simulink model "VTOLAutopilotController"  (R2025a)
settings: configuration reference "VTOLConfiguration" (kept outside this file)
undefined symbols (not defined in the file): Back_Transition_Rate, const, control, controlParams, ControlSampleTime, CriticalTiltAngle, DiscIntNeverNeededParam, dspblkCoreblockFVToolHelper, Fading_time, flightState, FSState, FWControlParams, FWTrimSpeed, gcbh, HoverMission, ReferenceFilterDen, ReferenceFilterNum, tilt_max, tiltIni, TransitioncontrolGains, uavParam, uavParams, VTOLcontrolGains, w_trim, WindDownRate
libraries: simulink x43, slpidlib x35, uavalgslib x7, simulink_extras x1
(part 2 of 8)

== system VTOLAutopilotController/Low level controller/Scheduler/Subsystem ==
  note: Multicopter Control Mixer
  note: MotorCommand1 : commanded phi torque (roll)
      | MotorCommand2 : commanded theta torque (pitch)
      | MotorCommand3 : commanded psi torque (yaw)
      | MotorCommand4 : commaned thrust
      | MotorCommand5 : command tilt
  FlightState : Inport
  FixedWingActuators : Inport  Port=2
  MotorCommands : Inport  Port=3
  TiltSchedule : Inport  Port=4
  TransitionDone : Inport  Port=5
  States : Inport  Port=6
  Actuator To Voltage : Subsystem
  Bus Selector1 : BusSelector  OutputSignals=Vb
  Merge : Merge  Inputs=4
  Scope{,1..3} (4 alike) : Scope
      Scope settings: ActiveDisplayYMinimum=-3975.75811  ActiveDisplayYMaximum=34801.34103  DataLoggingVariableName=ScopeData3
      Scope1 settings: ActiveDisplayYMinimum=0.5844  ActiveDisplayYMaximum=0.95477  DataLoggingVariableName=ScopeData4
      Scope2 settings: ActiveDisplayYMinimum=0.36457  ActiveDisplayYMaximum=0.73494  DataLoggingVariableName=ScopeData5
      Scope3 settings: ActiveDisplayYMinimum=0.36457  ActiveDisplayYMaximum=0.73494  DataLoggingVariableName=ScopeData6
  Switch Case : SwitchCase  CaseConditions={flightState.Hover, flightState.Transition, flightState.FixedWing,flightState.BackTransition}  ShowDefaultCase=off
  Switch Case Action Subsystem : Subsystem  TreatAsAtomicUnit=on
  Switch Case Action Subsystem1 : Subsystem  TreatAsAtomicUnit=on
  Switch Case Action Subsystem2 : Subsystem  TreatAsAtomicUnit=on
  Switch Case Action Subsystem3 : Subsystem  TreatAsAtomicUnit=on
  To Workspace : ToWorkspace  VariableName=Body_Velocity  SaveFormat=Timeseries  SampleTime=-1
  ActuatorControls : Outport  OutDataTypeStr=Bus: RotorCtrlBus
  wires:
  Merge/1 -> Scope/1, Actuator To Voltage/1(Motor Commands)
  Switch Case/4 -> Switch Case Action Subsystem3/Action
  MotorCommands/1 -> Switch Case Action Subsystem3/1(MixerCommands), Scope2/1, Switch Case Action Subsystem/1(MixerCommands), Switch Case Action Subsystem1/2(MixerCommands)
  States/1 -> Switch Case Action Subsystem1/5(State), Switch Case Action Subsystem2/3(State), Bus Selector1/1
  Switch Case Action Subsystem2/1(Actuator) -> Merge/3
  Switch Case Action Subsystem/1(Actuator) -> Merge/1
  Switch Case Action Subsystem3/1(Actuator) -> Merge/4
  FixedWingActuators/1 -> Switch Case Action Subsystem3/3(FixedWing), Switch Case Action Subsystem2/1(FixedWingCtrlBus), Switch Case Action Subsystem1/3(FixedWing)
  Switch Case/3 -> Switch Case Action Subsystem2/Action
  TransitionDone/1 -> Switch Case Action Subsystem1/4(TransitionDone), Switch Case Action Subsystem2/2(TransitionDone)
  Actuator To Voltage/1(To PWM) -> Scope1/1, ActuatorControls/1
  Switch Case/2 -> Switch Case Action Subsystem1/Action
  Switch Case Action Subsystem1/1(Actuator) -> Merge/2
  TiltSchedule/1 -> Switch Case Action Subsystem1/1(TiltSchedule), Switch Case Action Subsystem3/2(TiltSchedule)
  Switch Case/1 -> Switch Case Action Subsystem/Action
  Bus Selector1/1 -> To Workspace/1, Scope3/1  "<Vb>"
  FlightState/1 -> Switch Case/1

== system VTOLAutopilotController/Low level controller/Tilt Scheduler/Back Transition Scheduler ==
  Tilt Schedule : Inport
  FlightMode : Inport  Port=2
  States : Inport  Port=3
  Add : Sum  Commented=on  Inputs=+-
  Bus Selector : BusSelector  Commented=on  OutputSignals=Vb
  Constant1 : Constant  Value=flightState.BackTransition
  Constant2 : Constant  Value=0
  Constant5 : Constant  Value=-Back_Transition_Rate
  Constant6 : Constant  Commented=on  Value=4
  Discrete-Time Integrator : DiscreteIntegrator  ExternalReset=rising  InitialConditionSource=external  SampleTime=-1  LimitOutput=on  UpperSaturationLimit=pi/2  LowerSaturationLimit=0  ICPrevOutput=DiscIntNeverNeededParam  ICPrevScaledInput=DiscIntNeverNeededParam
  Equal : RelationalOperator  Operator===  OutDataTypeStr=boolean  RndMeth=Simplest  InputSameDT=off
  Saturation : Saturate  Commented=on  UpperLimit=pi/4  LowerLimit=-pi/4
  Selector : Selector  Commented=on  InputPortWidth=3  IndexOptions=Index vector (dialog)  Indices=[1]  OutputSizes=1
  Switch1 : Switch  Criteria=u2 > Threshold  SaturateOnIntegerOverflow=off  InputSameDT=off
  Switch2 : Switch  Threshold=1  SaturateOnIntegerOverflow=off  InputSameDT=off
  Vx Controller : slpidlib/PID Controller  Commented=on  Controller=P  Form=Parallel  TimeDomain=Discrete-time  UseExternalTs=off  SampleTime=0.005  IntegratorMethod=Forward Euler  FilterMethod=Forward Euler  ControllerParametersSource=internal  P=controlParams.P_BACK  I=0  UseKiTs=off  D=0.0379422021775223  UseExternalDerivativeSource=off  N=1.96946409823213  UseFilter=on  TunerSelectOption=Transfer Function Based (PID Tuner App)  InitialConditionSource=internal  InitialConditionForIntegrator=0  InitialConditionForFilter=0  DifferentiatorICPrevScaledInput=0  ExternalReset=none  TrackingMode=off  Kt=1  LimitOutput=off  SatLimitsSource=internal  UpperSaturationLimit=inf  LowerSaturationLimit=-inf  LinearizeAsGain=on  AntiWindupMode=none  Kb=1  LimitIntegrator=off  UpperIntegratorSaturationLimit=inf  LowerIntegratorSaturationLimit=-inf  POutMin=[]  POutMax=[]  IOutMin=[]  IOutMax=[]  DOutMin=[]  DOutMax=[]  NOutMin=[]  NOutMax=[]  SumOutMin=[]  SumOutMax=[]  SaturationOutMin=[]  SaturationOutMax=[]  PParamMin=[]  PParamMax=[]  IParamMin=[]  IParamMax=[]  DParamMin=[]  DParamMax=[]  NParamMin=[]  NParamMax=[]  KbParamMin=[]  KbParamMax=[]  KtParamMin=[]  KtParamMax=[]  KbOutMin=[]  KbOutMax=[]  KtOutMin=[]  KtOutMax=[]  IntegratorOutMin=[]  IntegratorOutMax=[]  FilterOutMin=[]  FilterOutMax=[]  SumI1OutMin=[]  SumI1OutMax=[]  SumI2OutMin=[]  SumI2OutMax=[]  SumI3OutMin=[]  SumI3OutMax=[]  SumI4OutMin=[]  SumI4OutMax=[]  SumDOutMin=[]  SumDOutMax=[]  DifferentiatorOutMin=[]  DifferentiatorOutMax=[]  FilterDiffOutCoefMin=[]  FilterDiffOutCoefMax=[]  ReciprocalOutMin=[]  ReciprocalOutMax=[]  SumDenOutMin=[]  SumDenOutMax=[]  SumNumOutMin=[]  SumNumOutMax=[]  DivideOutMin=[]  DivideOutMax=[]  UdiffTsProdOutMin=[]  UdiffTsProdOutMax=[]  NTsProdOutMin=[]  NTsProdOutMax=[]  UintegralTsProdOutMin=[]  UintegralTsProdOutMax=[]  UngainTsProdOutMin=[]  UngainTsProdOutMax=[]  ClampingZeroOutDataTypeStr=Inherit: Inherit via back propagation  ClampingZeroOutMin=[]  ClampingZeroOutMax=[]  FilterDenConstantOutDataTypeStr=Inherit: Inherit via back propagation  FilterDenConstantOutMin=[]  FilterDenConstantOutMax=[]  PCopyOutDataTypeStr=Inherit: Inherit via back propagation  PCopyOutMin=[]  PCopyOutMax=[]  NCopyOutDataTypeStr=Inherit: Inherit via back propagation  NCopyOutMin=[]  NCopyOutMax=[]  IntegratorContinuousStateAttributes=''  IntegratorStateMustResolveToSignalObject=off  IntegratorRTWStateStorageClass=Auto  FilterContinuousStateAttributes=''  FilterStateMustResolveToSignalObject=off  FilterRTWStateStorageClass=Auto  ParallelPVariant=InternalParameters  IdealPVariant=Disabled  IVariant=Disabled  DVariant=Disabled  IntegratorVariant=Disabled  SatVariant=Disabled  AWVariant=Disabled  PCopyVariant=Disabled  TRVariant=Disabled  FdbkBlocksVariant=Forward  IdealPFdbkVariant=Disabled  SatFdbkVariant=Disabled  DerivativeFilterVariant=Disabled  NVariant=Disabled  NCopyVariant=Disabled_SignalSpec  FilterICVariant=Disabled  IntegratorICVariant=Disabled  ExternalResetVariant=Disabled  TRSumVariant=Passthrough  SumFdbkVariant=Disabled  SumVariant=Passthrough_P  TsampFilterVariant=InternalTs  TsampNgainVariant=Passthrough  TsampIntegralVariant=Disabled_SignalSpec  ExternalSaturationOutDataTypeStr=Inherit: Same as second input  DerivativeSourceVariant=Disabled  PreIntVariant=InternalPreInt
  TiltAngle : Outport
  tag scope: BackTransitionFlag=global
  wires:
  States/1 -> Bus Selector/1
  Add/1 -> Vx Controller/1
  [BackTransitionFlag] -> Switch2/2
  Bus Selector/1 -> Selector/1  "<Vb>"
  Constant6/1 -> Add/1
  Selector/1 -> Add/2
  Vx Controller/1 -> Saturation/1
  Tilt Schedule/1 -> Switch2/3, Discrete-Time Integrator/3
  Switch2/1 -> TiltAngle/1
  Equal/1 -> [BackTransitionFlag]
  Constant1/1 -> Equal/1
  FlightMode/1 -> Equal/2
  Constant2/1 -> Switch1/3
  Switch1/1 -> Discrete-Time Integrator/1
  Constant5/1 -> Switch1/1
  [BackTransitionFlag] -> Discrete-Time Integrator/2, Switch1/2
  Discrete-Time Integrator/1 -> Switch2/1

== system VTOLAutopilotController/Low level controller/Tilt Scheduler/Forward Transition Scheduler ==
  FlightMode : Inport
  Constant : Constant  Value=pi/2
  Constant2 : Constant  Value=0
  Constant3 : Constant  Value=controlParams.CriticalTiltAngle
  Constant4 : Constant  Value=flightState.Transition
  Constant5 : Constant  Value=controlParams.TiltScheduleRate
  Discrete-Time Integrator : DiscreteIntegrator  ExternalReset=rising  SampleTime=-1  LimitOutput=on  UpperSaturationLimit=pi/2  LowerSaturationLimit=0  ICPrevOutput=DiscIntNeverNeededParam  ICPrevScaledInput=DiscIntNeverNeededParam
  Equal : RelationalOperator  Operator===  OutDataTypeStr=boolean  RndMeth=Simplest  InputSameDT=off
  LessThanOrEqual : RelationalOperator  Operator=<=  OutDataTypeStr=boolean  RndMeth=Simplest  InputSameDT=off
  Switch : Switch  Criteria=u2 > Threshold  SaturateOnIntegerOverflow=off  InputSameDT=off
  Switch1 : Switch  Criteria=u2 > Threshold  SaturateOnIntegerOverflow=off  InputSameDT=off
  FlightState : Outport
  Tilt Schedule : Outport  Port=2
  tag scope: ModeFlag=global
  wires:
  FlightMode/1 -> FlightState/1, Equal/2
  [ModeFlag] -> Discrete-Time Integrator/2, Switch1/2
  Discrete-Time Integrator/1 -> Switch/1, LessThanOrEqual/1
  LessThanOrEqual/1 -> Switch/2
  Equal/1 -> [ModeFlag]
  Constant3/1 -> LessThanOrEqual/2
  Switch1/1 -> Discrete-Time Integrator/1
  Constant5/1 -> Switch1/1
  Constant2/1 -> Switch1/3
  Constant4/1 -> Equal/1
  Constant/1 -> Switch/3
  Switch/1 -> Tilt Schedule/1

== system VTOLAutopilotController/Guidance Test Bench/ControlType/Guidance Testbench/Control Rate Transition ==
  "HoverSP " : Inport
  VTOLSP : Inport  Port=2
  FixedWingSP : Inport  Port=3
  AACSP : Inport  Port=4
  CtrlMode : Inport  Port=5
  FlightMode : Inport  Port=6
  Rate Transition{,1..3,5} (5 alike) : RateTransition  OutPortSampleTime=controlParams.ControlSampleTime
  Rate Transition4 : RateTransition  InitialCondition=flightState.Hover  OutPortSampleTime=controlParams.ControlSampleTime
  hoverSP : Outport
  vtolSP : Outport  Port=2
  fixedwingSP : Outport  Port=3
  aacSP : Outport  Port=4
  ctrlMode : Outport  Port=5
  flightMode : Outport  Port=6
  wires:
  AACSP/1 -> Rate Transition3/1
  VTOLSP/1 -> Rate Transition1/1
  Rate Transition5/1 -> ctrlMode/1
  CtrlMode/1 -> Rate Transition5/1
  Rate Transition3/1 -> aacSP/1
  "HoverSP "/1 -> Rate Transition/1
  Rate Transition1/1 -> vtolSP/1
  FixedWingSP/1 -> Rate Transition2/1
  Rate Transition2/1 -> fixedwingSP/1
  Rate Transition/1 -> hoverSP/1
  Rate Transition4/1 -> flightMode/1
  FlightMode/1 -> Rate Transition4/1

== system VTOLAutopilotController/Guidance Test Bench/ControlType/Guidance Testbench/Guidance Logic ==
  UAVState : Inport
  GCSCommands : Inport  Port=2
  Ground : Inport  Port=3
  Atan2 : Trigonometry  Operator=atan2
  Bus Creator : BusCreator  Commented=on  Inputs=4
  Bus Selector1 : BusSelector  OutputSignals=x,y,z,vy,vx
  Demux : Demux  Commented=on
  Guidance Stateflow : Subsystem
  Interface : Subsystem
  Mux : Mux
  Mux2 : Mux  Inputs=2
  Subsystem : Subsystem
  Terminator : Terminator
  HoverSP : Outport
  VTOLSP : Outport  Port=2
  FixedWingSP : Outport  Port=3
  AACSP : Outport  Port=4
  CtrlMode : Outport  Port=5
  FlightMode : Outport  Port=6
  wires:
  Mux/1 -> Guidance Stateflow/1(Pose)
  Bus Selector1/5 -> Atan2/2  "<vx>"
  GCSCommands/1 -> Guidance Stateflow/2(GCSCommands)
  Bus Selector1/4 -> Atan2/1  "<vy>"
  Bus Selector1/3 -> Mux2/2, Mux/3  "<z>"
  Bus Selector1/2 -> Mux/2  "<y>"
  UAVState/1 -> Subsystem/1(UAVState), Interface/1(UAVState)
  Bus Selector1/1 -> Mux/1  "<x>"
  Interface/1(States) -> Bus Selector1/1
  Demux/3 -> Bus Creator/3  "Z"
  Demux/1 -> Bus Creator/1  "X"
  Demux/2 -> Bus Creator/2  "Y"
  Mux2/1 -> Guidance Stateflow/3(LandingStates)
  Atan2/1 -> Mux2/1, Mux/4
  Subsystem/1(States) -> Guidance Stateflow/4(States)
  Guidance Stateflow/4(FixedWingSP) -> FixedWingSP/1
  Guidance Stateflow/3(AACSP) -> AACSP/1
  Guidance Stateflow/5(CtrlMode) -> CtrlMode/1
  Guidance Stateflow/6(FlightMode) -> FlightMode/1
  Demux/4 -> Bus Creator/4  "Yaw"
  Ground/1 -> Guidance Stateflow/5(Ground)
  Guidance Stateflow/1(HoverSP) -> HoverSP/1
  Guidance Stateflow/2(VTOLSP) -> VTOLSP/1
  Guidance Stateflow/7(GuidanceMode) -> Terminator/1

== system VTOLAutopilotController/Guidance Test Bench/ControlType/Manual Control/Command Interface ==
  note: Limit rate for Manual control to keep Flight in operational envelope
  BusElementIn : Inport  PortName=Global Mission  Element=position
  BusElementIn1 : Inport  PortName=Global Mission  Element=params
  Aircraft States : Inport  Port=2
  Basic Control  Switching : Stateflow chart  TreatAsAtomicUnit=on
  Bus Creator : BusCreator  Inputs=5  OutDataTypeStr=Bus: AAC
  Bus Creator1 : BusCreator  Inputs=4  OutDataTypeStr=Bus: FixedWingCommandBus
  Bus Creator2 : BusCreator  Inputs=4
  Constant{,1..2,5..6} (5 alike) : Constant  Value=0
  Constant4 : Constant  Value=25
  Control Rate Transition : Subsystem
  Data Type Conversion : DataTypeConversion  OutDataTypeStr=Enum: flightState  SaturateOnIntegerOverflow=off  RndMeth=Floor
  Data Type Conversion1 : DataTypeConversion  OutDataTypeStr=uint8  SaturateOnIntegerOverflow=off  RndMeth=Floor
  Degrees to Radians : simulink_extras/Transformations/Degrees to Radians
  Demux : Demux  Outputs=3
  Demux1 : Demux
  Gain : Gain  Gain=-1
  Rate Limiter : RateLimiter  RisingSlewLimit=3  FallingSlewLimit=-3  SampleTimeMode=inherited
  Round : Rounding  Operator=round
  Subsystem : Subsystem
  ctrlMode : Outport
  FixedWingSP : Outport  Port=2
  AACSP : Outport  Port=3
  PositionCmds : Outport  Port=4
  FlightMode : Outport  Port=5
  wires:
  Demux1/3 -> Bus Creator/2  "altitude"
  Bus Creator2/1 -> Control Rate Transition/5(Position)
  Constant5/1 -> Bus Creator/5  "climbrate"
  Demux1/4 -> Degrees to Radians/1
  Bus Creator/1 -> Control Rate Transition/4(AACSetpoint)
  Demux/3 -> Gain/1  "Z"
  Data Type Conversion/1 -> Basic Control  Switching/1(FlightMode), Control Rate Transition/1(FM)
  Constant/1 -> Bus Creator1/1  "roll"
  Bus Creator1/1 -> Control Rate Transition/3(FixedWingSetpoint)
  Constant1/1 -> Bus Creator1/2  "pitch"
  Constant4/1 -> Bus Creator/4  "L1"
  Constant2/1 -> Bus Creator1/3  "yaw"
  Demux1/2 -> Bus Creator/1, Bus Creator1/4  "airspeed"
  Control Rate Transition/2(FixedWingSP) -> FixedWingSP/1
  Degrees to Radians/1 -> Bus Creator/3  "course"
  Demux/1 -> Bus Creator2/1  "X"
  Aircraft States/1 -> Subsystem/1(UAVState)
  Demux/2 -> Bus Creator2/2  "Y"
  Gain/1 -> Rate Limiter/1  "Z"
  Basic Control  Switching/1(controlMode) -> Control Rate Transition/2("ControlMode ")
  Control Rate Transition/1(ctrlMode) -> ctrlMode/1
  Control Rate Transition/3(AACSP) -> AACSP/1
  Control Rate Transition/4(PositionCmds) -> PositionCmds/1
  Control Rate Transition/5(FlightMode) -> FlightMode/1
  Demux1/1 -> Round/1
  Subsystem/1(States) -> Basic Control  Switching/2(States)
  Constant6/1 -> Bus Creator2/4
  Rate Limiter/1 -> Bus Creator2/3  "Z"
  BusElementIn/1 -> Demux/1
  BusElementIn1/1 -> Demux1/1
  Round/1 -> Data Type Conversion1/1
  Data Type Conversion1/1 -> Data Type Conversion/1

== system VTOLAutopilotController/Guidance Test Bench/Variant Subsystem/Reference Tracking /Fixed Wing Reference ==
  AAC Commands : Inport
  States : Inport  Port=2
  Bus Creator1 : BusCreator  Inputs=2
  Bus Creator2 : BusCreator  Inputs=3
  Bus Selector : BusSelector  OutputSignals=airspeed,Xe,course
  Bus Selector3 : BusSelector  OutputSignals=airspeed,altitude,course
  Gain : Gain  Gain=-1
  Mux1 : Mux  Inputs=3
  Selector : Selector  InputPortWidth=3  IndexOptions=Index vector (dialog)  Indices=3  OutputSizes=1
  To Workspace1 : ToWorkspace  VariableName=FixedWingCmdFdbk  SaveFormat=Structure With Time  SampleTime=-1
  wires:
  Selector/1 -> Gain/1
  Bus Selector3/1 -> Mux1/1  "<airspeed>"
  Bus Selector/1 -> Bus Creator2/1  "<airspeed>"
  Bus Selector3/2 -> Mux1/2  "<altitude>"
  Bus Selector/3 -> Bus Creator2/3  "<course>"
  Mux1/1 -> Bus Creator1/1
  Bus Creator1/1 -> To Workspace1/1
  Bus Selector3/3 -> Mux1/3  "<course>"
  Gain/1 -> Bus Creator2/2  "altitude"
  Bus Creator2/1 -> Bus Creator1/2
  AAC Commands/1 -> Bus Selector3/1
  Bus Selector/2 -> Selector/1  "<Xe>"
  States/1 -> Bus Selector/1

== system VTOLAutopilotController/Guidance Test Bench/Variant Subsystem/Reference Tracking /Hover Reference ==
  Position Command : Inport
  Position Reference : Inport  Port=2
  Bus Creator : BusCreator  Inputs=2
  Bus Selector : BusSelector  OutputSignals=localposition
  Bus Selector1 : BusSelector  OutputSignals=Xe  OutputAsBus=on
  Demux : Demux  Outputs=3
  Mux : Mux  Inputs=3
  To Workspace : ToWorkspace  VariableName=PositionCmdFdbk  SaveFormat=Structure With Time  SampleTime=-1
  wires:
  Position Reference/1 -> Bus Selector1/1
  Bus Selector1/1 -> Bus Creator/2
  Bus Creator/1 -> To Workspace/1
  Mux/1 -> Bus Creator/1
  Position Command/1 -> Bus Selector/1
  Bus Selector/1 -> Demux/1  "<localposition>"
  Demux/1 -> Mux/1
  Demux/2 -> Mux/2
  Demux/3 -> Mux/3

== system VTOLAutopilotController/Guidance Test Bench/Variant Subsystem/Reference Tracking /Transition Reference ==
  States : Inport
  Bus Creator : BusCreator  Inputs=4
  Bus Selector4 : BusSelector  OutputSignals=airspeed,RotorParameters.Tilt1,Euler,Xe
  Gain : Gain  Gain=-1
  Selector : Selector  InputPortWidth=3  IndexOptions=Index vector (dialog)  Indices=[2]  OutputSizes=1
  Selector1 : Selector  InputPortWidth=3  IndexOptions=Index vector (dialog)  Indices=[3]  OutputSizes=1
  To Workspace1 : ToWorkspace  VariableName=TransitionFeedback  SaveFormat=Structure With Time  SampleTime=-1
  wires:
  States/1 -> Bus Selector4/1
  Bus Selector4/3 -> Selector/1  "<Euler>"
  Bus Selector4/4 -> Selector1/1  "<Xe>"
  Selector1/1 -> Gain/1
  Bus Selector4/1 -> Bus Creator/1  "<airspeed>"
  Selector/1 -> Bus Creator/3  "pitch"
  Gain/1 -> Bus Creator/4  "altitude"
  Bus Creator/1 -> To Workspace1/1
  Bus Selector4/2 -> Bus Creator/2  "<Tilt1>"

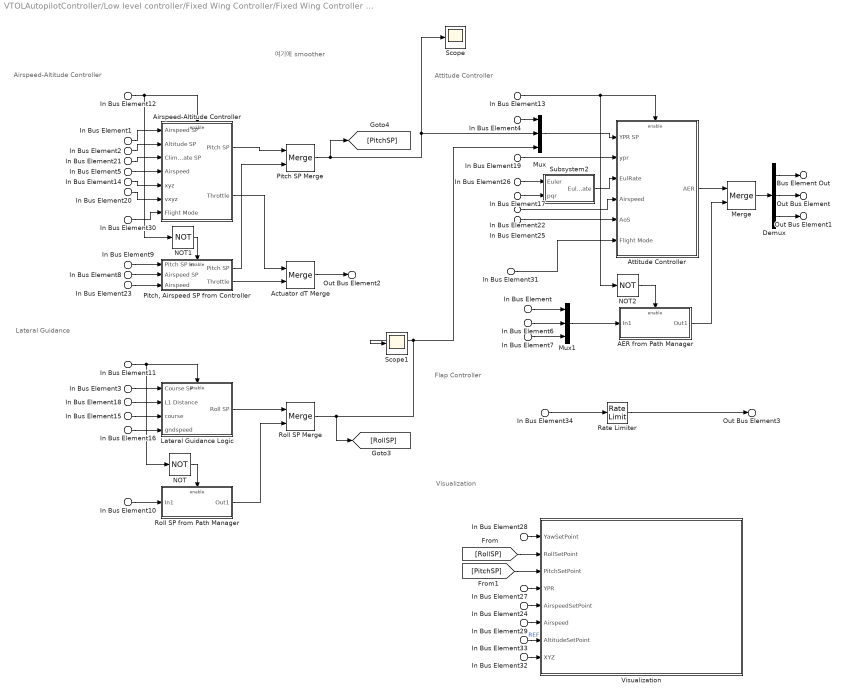
== system VTOLAutopilotController/Low level controller/Fixed Wing Controller/Fixed Wing Controller Module/Fixed Wing Controller Simulation ==
  note: 여기에 smoother
  note: Attitude Controller
  note: Lateral Guidance
  note: Airspeed-Altitude Controller
  note: Visualization
  note: Flap Controller
  In Bus Element14 : Inport  PortName=States  Element=Xe
  In Bus Element32 : Inport  PortName=States  Element=Xe
  In Bus Element15 : Inport  PortName=States  Element=course
  In Bus Element17 : Inport  PortName=States  Element=pqr
  In Bus Element{5,22..23,29} (4 alike) : Inport  PortName=States  Element=airspeed
  In Bus Element19 : Inport  PortName=States  Element=ypr
  In Bus Element27 : Inport  PortName=States  Element=ypr
  In Bus Element16 : Inport  PortName=States  Element=gndspeed
  In Bus Element26 : Inport  PortName=States  Element=Euler
  In Bus Element20 : Inport  PortName=States  Element=Ve
  In Bus Element25 : Inport  PortName=States  Element=aos
  In Bus Element11 : Inport  Port=2  PortName=Control Mode  Element=lateralguidance
  In Bus Element12 : Inport  Port=2  PortName=Control Mode  Element=airspeedaltitude
  In Bus Element13 : Inport  Port=2  PortName=Control Mode  Element=attitude
  In Bus Element1 : Inport  Port=3  PortName=AAC SP  Element=airspeed
  In Bus Element24 : Inport  Port=3  PortName=AAC SP  Element=airspeed
  In Bus Element2 : Inport  Port=3  PortName=AAC SP  Element=altitude
  In Bus Element33 : Inport  Port=3  PortName=AAC SP  Element=altitude
  In Bus Element18 : Inport  Port=3  PortName=AAC SP  Element=L1
  In Bus Element21 : Inport  Port=3  PortName=AAC SP  Element=course
  In Bus Element3 : Inport  Port=3  PortName=AAC SP  Element=course
  In Bus Element4 : Inport  Port=4  PortName=FixedWingSP  Element=yaw
  In Bus Element28 : Inport  Port=4  PortName=FixedWingSP  Element=yaw
  In Bus Element9 : Inport  Port=4  PortName=FixedWingSP  Element=pitch
  In Bus Element10 : Inport  Port=4  PortName=FixedWingSP  Element=roll
  In Bus Element8 : Inport  Port=4  PortName=FixedWingSP  Element=airspeed
  In Bus Element34 : Inport  Port=4  PortName=FixedWingSP  Element=flap
  In Bus Element : Inport  Port=5  PortName=AERT  Element=aileron
  In Bus Element6 : Inport  Port=5  PortName=AERT  Element=elevator
  In Bus Element7 : Inport  Port=5  PortName=AERT  Element=rudder
  In Bus Element30 : Inport  Port=6  PortName=Flight Mode
  In Bus Element31 : Inport  Port=6  PortName=Flight Mode
  AER from Path Manager : Subsystem  TreatAsAtomicUnit=on
  Actuator dT Merge : Merge
  Airspeed-Altitude Controller : Subsystem
  Attitude Controller : Subsystem
  Demux : Demux  Outputs=3
  Lateral Guidance Logic : Subsystem
  Merge : Merge
  Mux : Mux  Inputs=3
  Mux1 : Mux  Inputs=3
  NOT : Logic  Operator=NOT  IconShape=distinctive  AllPortsSameDT=off  OutDataTypeStr=boolean
  NOT1 : Logic  Operator=NOT  IconShape=distinctive  AllPortsSameDT=off  OutDataTypeStr=boolean
  NOT2 : Logic  Operator=NOT  IconShape=distinctive  AllPortsSameDT=off  OutDataTypeStr=boolean
  Pitch SP Merge : Merge
  "Pitch, Airspeed SP from Controller" : Subsystem  TreatAsAtomicUnit=on
  Rate Limiter : RateLimiter  RisingSlewLimit=controlParams.FWmaxFlapSlewrate  FallingSlewLimit=controlParams.FWminFlapSlewrate  SampleTimeMode=inherited
  Roll SP Merge : Merge
  Roll SP from Path Manager : Subsystem  TreatAsAtomicUnit=on
  Scope : Scope
      settings: ActiveDisplayYMinimum=-0.1996  ActiveDisplayYMaximum=0.41003  DataLoggingVariableName=ScopeData5
  Scope1 : Scope
      settings: ActiveDisplayYMinimum=-0.90942  ActiveDisplayYMaximum=0.85994  DataLoggingVariableName=ScopeData2
  Subsystem2 : Subsystem
  Visualization : Subsystem  Variant=on  VariantControl=Visualization
  Bus Element Out : Outport  PortName=Actuator  Element=dA
  Out Bus Element : Outport  PortName=Actuator  Element=dE
  Out Bus Element1 : Outport  PortName=Actuator  Element=dR
  Out Bus Element2 : Outport  PortName=Actuator  Element=dT
  Out Bus Element3 : Outport  PortName=Actuator  Element=dF
  wires:
  Pitch SP Merge/1 -> Scope/1, Mux/2, [PitchSP]
  Demux/2 -> Out Bus Element/1
  Airspeed-Altitude Controller/1(Pitch SP) -> Pitch SP Merge/1
  In Bus Element18/1 -> Lateral Guidance Logic/2(L1 Distance)
  In Bus Element1/1 -> Airspeed-Altitude Controller/1(Airspeed SP)
  In Bus Element17/1 -> Subsystem2/2(pqr)
  Actuator dT Merge/1 -> Out Bus Element2/1
  In Bus Element26/1 -> Subsystem2/1(Euler)
  In Bus Element11/1 -> Lateral Guidance Logic/Enable, NOT/1
  Subsystem2/1(Euler Rate) -> Attitude Controller/3(EulRate)
  In Bus Element13/1 -> NOT2/1, Attitude Controller/Enable
  In Bus Element3/1 -> Lateral Guidance Logic/1(Course SP)
  In Bus Element22/1 -> Attitude Controller/4(Airspeed)
  Demux/3 -> Out Bus Element1/1
  Roll SP from Path Manager/1(Out1) -> Roll SP Merge/2
  In Bus Element4/1 -> Mux/1
  In Bus Element14/1 -> Airspeed-Altitude Controller/5(xyz)
  In Bus Element15/1 -> Lateral Guidance Logic/3(course)
  In Bus Element6/1 -> Mux1/2
  Mux1/1 -> AER from Path Manager/1(In1)
  Airspeed-Altitude Controller/2(Throttle) -> Actuator dT Merge/1
  "Pitch, Airspeed SP from Controller"/1(Pitch SP) -> Pitch SP Merge/2
  In Bus Element16/1 -> Lateral Guidance Logic/4(gndspeed)
  "Pitch, Airspeed SP from Controller"/2(Throttle) -> Actuator dT Merge/2
  In Bus Element/1 -> Mux1/1
  In Bus Element2/1 -> Airspeed-Altitude Controller/2(Altitude SP)
  In Bus Element7/1 -> Mux1/3
  In Bus Element9/1 -> "Pitch, Airspeed SP from Controller"/1(Pitch SP In)
  Merge/1 -> Demux/1
  In Bus Element10/1 -> Roll SP from Path Manager/1(In1)
  Mux/1 -> Attitude Controller/1(YPR SP)
  Attitude Controller/1(AER) -> Merge/1
  NOT1/1 -> "Pitch, Airspeed SP from Controller"/Enable
  In Bus Element8/1 -> "Pitch, Airspeed SP from Controller"/2(Airspeed SP)
  In Bus Element20/1 -> Airspeed-Altitude Controller/6(vxyz)
  In Bus Element19/1 -> Attitude Controller/2(ypr)
  NOT2/1 -> AER from Path Manager/Enable
  In Bus Element23/1 -> "Pitch, Airspeed SP from Controller"/3(Airspeed)
  Lateral Guidance Logic/1(Roll SP) -> Roll SP Merge/1
  NOT/1 -> Roll SP from Path Manager/Enable
  AER from Path Manager/1(Out1) -> Merge/2
  In Bus Element5/1 -> Airspeed-Altitude Controller/4(Airspeed)
  Demux/1 -> Bus Element Out/1
  In Bus Element21/1 -> Airspeed-Altitude Controller/3(Climb Rate SP)
  Roll SP Merge/1 -> [RollSP], Mux/3, Scope1/1
  In Bus Element12/1 -> Airspeed-Altitude Controller/Enable, NOT1/1
  In Bus Element28/1 -> Visualization/1(YawSetPoint)
  In Bus Element27/1 -> Visualization/4(YPR)
  In Bus Element24/1 -> Visualization/5(AirspeedSetPoint)
  In Bus Element29/1 -> Visualization/6(Airspeed)
  In Bus Element33/1 -> Visualization/7(AltitudeSetPoint)  "REF"
  In Bus Element32/1 -> Visualization/8(XYZ)
  [RollSP] -> Visualization/2(RollSetPoint)
  [PitchSP] -> Visualization/3(PitchSetPoint)
  In Bus Element25/1 -> Attitude Controller/5(AoS)
  In Bus Element30/1 -> Airspeed-Altitude Controller/7(Flight Mode)
  In Bus Element31/1 -> Attitude Controller/6(Flight Mode)
  In Bus Element34/1 -> Rate Limiter/1
  Rate Limiter/1 -> Out Bus Element3/1

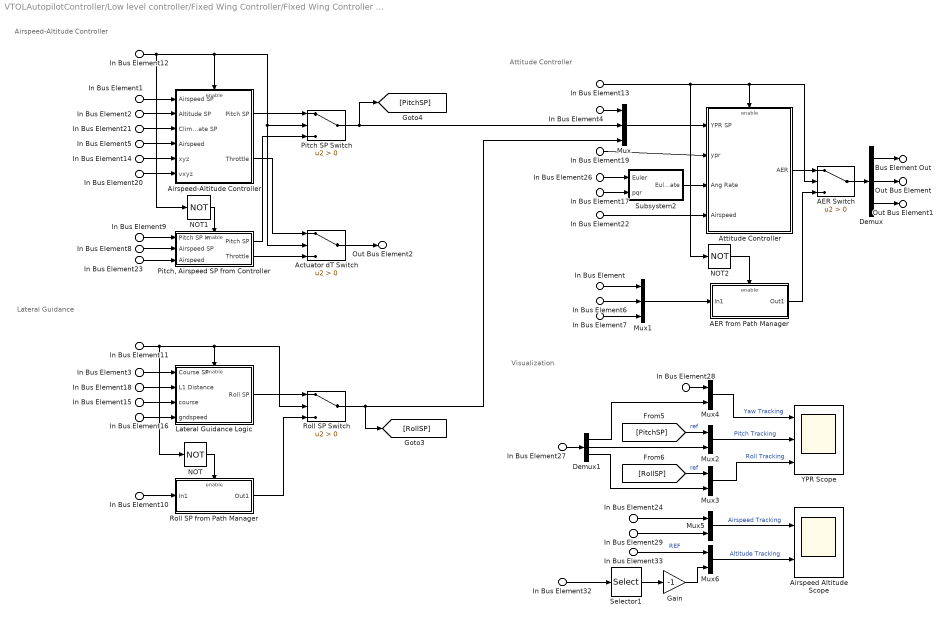
== system VTOLAutopilotController/Low level controller/Fixed Wing Controller/Fixed Wing Controller Module/Fixed Wing Controller Tuning ==
  note: Visualization
  note: Attitude Controller
  note: Airspeed-Altitude Controller
  note: Lateral Guidance
  In Bus Element14 : Inport  PortName=States  Element=Xe
  In Bus Element32 : Inport  PortName=States  Element=Xe
  In Bus Element15 : Inport  PortName=States  Element=course
  In Bus Element17 : Inport  PortName=States  Element=pqr
  In Bus Element{5,22..23,29} (4 alike) : Inport  PortName=States  Element=airspeed
  In Bus Element19 : Inport  PortName=States  Element=ypr
  In Bus Element27 : Inport  PortName=States  Element=ypr
  In Bus Element16 : Inport  PortName=States  Element=gndspeed
  In Bus Element26 : Inport  PortName=States  Element=Euler
  In Bus Element20 : Inport  PortName=States  Element=Ve_ground
  In Bus Element11 : Inport  Port=2  PortName=Control Mode  Element=lateralGuidance
  In Bus Element12 : Inport  Port=2  PortName=Control Mode  Element=airspeedAltitude
  In Bus Element13 : Inport  Port=2  PortName=Control Mode  Element=attitude
  In Bus Element1 : Inport  Port=3  PortName=AAC SP  Element=airspeed
  In Bus Element24 : Inport  Port=3  PortName=AAC SP  Element=airspeed
  In Bus Element2 : Inport  Port=3  PortName=AAC SP  Element=altitude
  In Bus Element33 : Inport  Port=3  PortName=AAC SP  Element=altitude
  In Bus Element18 : Inport  Port=3  PortName=AAC SP  Element=L1
  In Bus Element21 : Inport  Port=3  PortName=AAC SP  Element=course
  In Bus Element3 : Inport  Port=3  PortName=AAC SP  Element=course
  In Bus Element4 : Inport  Port=4  PortName=FixedWingSP  Element=yaw
  In Bus Element28 : Inport  Port=4  PortName=FixedWingSP  Element=yaw
  In Bus Element9 : Inport  Port=4  PortName=FixedWingSP  Element=pitch
  In Bus Element10 : Inport  Port=4  PortName=FixedWingSP  Element=roll
  In Bus Element8 : Inport  Port=4  PortName=FixedWingSP  Element=airspeed
  In Bus Element : Inport  Port=5  PortName=AERT  Element=aileron
  In Bus Element6 : Inport  Port=5  PortName=AERT  Element=elevator
  In Bus Element7 : Inport  Port=5  PortName=AERT  Element=rudder
  AER Switch : Switch  Criteria=u2 > Threshold  SaturateOnIntegerOverflow=off  InputSameDT=off
  AER from Path Manager : Subsystem  TreatAsAtomicUnit=on
  Actuator dT Switch : Switch  Criteria=u2 > Threshold  SaturateOnIntegerOverflow=off  InputSameDT=off
  Airspeed Altitude Scope : Scope  NumInputPorts=2
      settings: ActiveDisplayYMinimum=-2.71065  ActiveDisplayYMaximum=24.39589  DataLoggingVariableName=ScopeData3
  Airspeed-Altitude Controller : Subsystem
  Attitude Controller : Subsystem
  Demux : Demux  Outputs=3
  Demux1 : Demux  Outputs=3
  Gain : Gain  Gain=-1
  Lateral Guidance Logic : Subsystem
  Mux : Mux  Inputs=3
  Mux1 : Mux  Inputs=3
  Mux{2..6} (5 alike) : Mux  Inputs=2
  NOT : Logic  Operator=NOT  IconShape=distinctive  AllPortsSameDT=off  OutDataTypeStr=boolean
  NOT1 : Logic  Operator=NOT  IconShape=distinctive  AllPortsSameDT=off  OutDataTypeStr=boolean
  NOT2 : Logic  Operator=NOT  IconShape=distinctive  AllPortsSameDT=off  OutDataTypeStr=boolean
  Pitch SP Switch : Switch  Criteria=u2 > Threshold  SaturateOnIntegerOverflow=off  InputSameDT=off
  "Pitch, Airspeed SP from Controller" : Subsystem  TreatAsAtomicUnit=on
  Roll SP Switch : Switch  Criteria=u2 > Threshold  SaturateOnIntegerOverflow=off  InputSameDT=off
  Roll SP from Path Manager : Subsystem  TreatAsAtomicUnit=on
  Selector1 : Selector  InputPortWidth=3  IndexOptions=Index vector (dialog)  Indices=[3]  OutputSizes=1
  Subsystem2 : Subsystem
  YPR Scope : Scope  NumInputPorts=3
      settings: ActiveDisplayYMinimum=-1  ActiveDisplayYMaximum=1  DataLoggingVariableName=ScopeData2
  Bus Element Out : Outport  PortName=Actuator  Element=dA
  Out Bus Element : Outport  PortName=Actuator  Element=dE
  Out Bus Element1 : Outport  PortName=Actuator  Element=dR
  Out Bus Element2 : Outport  PortName=Actuator  Element=dT
  wires:
  Mux/1 -> Attitude Controller/1(YPR SP)
  Attitude Controller/1(AER) -> AER Switch/1
  AER Switch/1 -> Demux/1
  Demux/1 -> Bus Element Out/1
  NOT/1 -> Roll SP from Path Manager/Enable
  Lateral Guidance Logic/1(Roll SP) -> Roll SP Switch/1
  Roll SP from Path Manager/1(Out1) -> Roll SP Switch/3
  NOT1/1 -> "Pitch, Airspeed SP from Controller"/Enable
  In Bus Element8/1 -> "Pitch, Airspeed SP from Controller"/2(Airspeed SP)
  "Pitch, Airspeed SP from Controller"/1(Pitch SP) -> Pitch SP Switch/3
  Airspeed-Altitude Controller/2(Throttle) -> Actuator dT Switch/1
  "Pitch, Airspeed SP from Controller"/2(Throttle) -> Actuator dT Switch/3
  Mux1/1 -> AER from Path Manager/1(In1)
  AER from Path Manager/1(Out1) -> AER Switch/3
  NOT2/1 -> AER from Path Manager/Enable
  In Bus Element/1 -> Mux1/1
  In Bus Element6/1 -> Mux1/2
  In Bus Element7/1 -> Mux1/3
  In Bus Element9/1 -> "Pitch, Airspeed SP from Controller"/1(Pitch SP In)
  In Bus Element10/1 -> Roll SP from Path Manager/1(In1)
  In Bus Element11/1 -> Roll SP Switch/2, Lateral Guidance Logic/Enable, NOT/1
  In Bus Element18/1 -> Lateral Guidance Logic/2(L1 Distance)
  In Bus Element14/1 -> Airspeed-Altitude Controller/5(xyz)
  In Bus Element19/1 -> Attitude Controller/2(ypr)
  In Bus Element16/1 -> Lateral Guidance Logic/4(gndspeed)
  In Bus Element5/1 -> Airspeed-Altitude Controller/4(Airspeed)
  In Bus Element12/1 -> Actuator dT Switch/2, Pitch SP Switch/2, Airspeed-Altitude Controller/Enable, NOT1/1
  In Bus Element2/1 -> Airspeed-Altitude Controller/2(Altitude SP)
  Roll SP Switch/1 -> Mux/3, [RollSP]
  In Bus Element15/1 -> Lateral Guidance Logic/3(course)
  Demux/3 -> Out Bus Element1/1
  In Bus Element13/1 -> NOT2/1, AER Switch/2, Attitude Controller/Enable
  In Bus Element4/1 -> Mux/1
  In Bus Element22/1 -> Attitude Controller/4(Airspeed)
  In Bus Element3/1 -> Lateral Guidance Logic/1(Course SP)
  In Bus Element1/1 -> Airspeed-Altitude Controller/1(Airspeed SP)
  In Bus Element20/1 -> Airspeed-Altitude Controller/6(vxyz)
  In Bus Element21/1 -> Airspeed-Altitude Controller/3(Climb Rate SP)
  In Bus Element23/1 -> "Pitch, Airspeed SP from Controller"/3(Airspeed)
  In Bus Element27/1 -> Demux1/1
  Demux1/1 -> Mux4/2
  Demux1/2 -> Mux2/2
  Demux1/3 -> Mux3/2
  In Bus Element17/1 -> Subsystem2/2(pqr)
  In Bus Element26/1 -> Subsystem2/1(Euler)
  Subsystem2/1(Euler Rate) -> Attitude Controller/3(Ang Rate)
  Actuator dT Switch/1 -> Out Bus Element2/1
  Demux/2 -> Out Bus Element/1
  Pitch SP Switch/1 -> [PitchSP], Mux/2
  Airspeed-Altitude Controller/1(Pitch SP) -> Pitch SP Switch/1
  [PitchSP] -> Mux2/1  "ref"
  In Bus Element28/1 -> Mux4/1
  [RollSP] -> Mux3/1  "ref"
  Mux4/1 -> YPR Scope/1  "Yaw Tracking"
  Mux2/1 -> YPR Scope/2  "Pitch Tracking"
  Mux3/1 -> YPR Scope/3  "Roll Tracking"
  Mux5/1 -> Airspeed Altitude Scope/1  "Airspeed Tracking"
  Mux6/1 -> Airspeed Altitude Scope/2  "Altitude Tracking"
  In Bus Element24/1 -> Mux5/1
  In Bus Element29/1 -> Mux5/2
  In Bus Element32/1 -> Selector1/1
  Selector1/1 -> Gain/1
  Gain/1 -> Mux6/2
  In Bus Element33/1 -> Mux6/1  "REF"

== system VTOLAutopilotController/Low level controller/Multicopter Controller/Attitude & Altitude controller/Altitude Control ==
  note: Maintain altitude previously set when in transition
  States : Inport
  Z ref : Inport  Port=2
  InTransition : Inport  Port=3
  FlightMode : Inport  Port=4
  Alt signal condition : Subsystem
  Altitude controller : slpidlib/PID Controller  Controller=P  Form=Parallel  TimeDomain=Continuous-time  UseExternalTs=off  SampleTime=-1  IntegratorMethod=Forward Euler  FilterMethod=Forward Euler  ControllerParametersSource=internal  P=VTOLcontrolGains.P_Z  I=controlParams.I_Z  UseKiTs=off  D=controlParams.D_Z  UseExternalDerivativeSource=off  N=controlParams.N_Z  UseFilter=on  TunerSelectOption=Transfer Function Based (PID Tuner App)  InitialConditionSource=internal  InitialConditionForIntegrator=0  InitialConditionForFilter=0  DifferentiatorICPrevScaledInput=0  ExternalReset=none  TrackingMode=off  Kt=1  LimitOutput=off  SatLimitsSource=internal  UpperSaturationLimit=inf  LowerSaturationLimit=-inf  LinearizeAsGain=on  AntiWindupMode=none  Kb=1  LimitIntegrator=off  UpperIntegratorSaturationLimit=inf  LowerIntegratorSaturationLimit=-inf  POutMin=[]  POutMax=[]  IOutMin=[]  IOutMax=[]  DOutMin=[]  DOutMax=[]  NOutMin=[]  NOutMax=[]  SumOutMin=[]  SumOutMax=[]  SaturationOutMin=[]  SaturationOutMax=[]  PParamMin=[]  PParamMax=[]  IParamMin=[]  IParamMax=[]  DParamMin=[]  DParamMax=[]  NParamMin=[]  NParamMax=[]  KbParamMin=[]  KbParamMax=[]  KtParamMin=[]  KtParamMax=[]  KbOutMin=[]  KbOutMax=[]  KtOutMin=[]  KtOutMax=[]  IntegratorOutMin=[]  IntegratorOutMax=[]  FilterOutMin=[]  FilterOutMax=[]  SumI1OutMin=[]  SumI1OutMax=[]  SumI2OutMin=[]  SumI2OutMax=[]  SumI3OutMin=[]  SumI3OutMax=[]  SumI4OutMin=[]  SumI4OutMax=[]  SumDOutMin=[]  SumDOutMax=[]  DifferentiatorOutMin=[]  DifferentiatorOutMax=[]  FilterDiffOutCoefMin=[]  FilterDiffOutCoefMax=[]  ReciprocalOutMin=[]  ReciprocalOutMax=[]  SumDenOutMin=[]  SumDenOutMax=[]  SumNumOutMin=[]  SumNumOutMax=[]  DivideOutMin=[]  DivideOutMax=[]  UdiffTsProdOutMin=[]  UdiffTsProdOutMax=[]  NTsProdOutMin=[]  NTsProdOutMax=[]  UintegralTsProdOutMin=[]  UintegralTsProdOutMax=[]  UngainTsProdOutMin=[]  UngainTsProdOutMax=[]  ClampingZeroOutDataTypeStr=Inherit: Inherit via back propagation  ClampingZeroOutMin=[]  ClampingZeroOutMax=[]  FilterDenConstantOutDataTypeStr=Inherit: Inherit via back propagation  FilterDenConstantOutMin=[]  FilterDenConstantOutMax=[]  PCopyOutDataTypeStr=Inherit: Inherit via back propagation  PCopyOutMin=[]  PCopyOutMax=[]  NCopyOutDataTypeStr=Inherit: Inherit via back propagation  NCopyOutMin=[]  NCopyOutMax=[]  IntegratorContinuousStateAttributes=''  IntegratorStateMustResolveToSignalObject=off  IntegratorRTWStateStorageClass=Auto  FilterContinuousStateAttributes=''  FilterStateMustResolveToSignalObject=off  FilterRTWStateStorageClass=Auto  ParallelPVariant=InternalParameters  IdealPVariant=Disabled  IVariant=Disabled  DVariant=Disabled  IntegratorVariant=Disabled  SatVariant=Disabled  AWVariant=Disabled  PCopyVariant=Disabled  TRVariant=Disabled  FdbkBlocksVariant=Forward  IdealPFdbkVariant=Disabled  SatFdbkVariant=Disabled  DerivativeFilterVariant=Disabled  NVariant=Disabled  NCopyVariant=Disabled_SignalSpec  FilterICVariant=Disabled  IntegratorICVariant=Disabled  ExternalResetVariant=Disabled  TRSumVariant=Passthrough  SumFdbkVariant=Disabled  SumVariant=Passthrough_P  TsampFilterVariant=InternalTs  TsampNgainVariant=Passthrough  TsampIntegralVariant=Disabled_SignalSpec  ExternalSaturationOutDataTypeStr=Inherit: Same as second input  DerivativeSourceVariant=Disabled  PreIntVariant=InternalPreInt
  Altitude rate controller : slpidlib/PID Controller  Controller=PID  Form=Parallel  TimeDomain=Discrete-time  UseExternalTs=off  SampleTime=-1  IntegratorMethod=Forward Euler  FilterMethod=Forward Euler  ControllerParametersSource=internal  P=VTOLcontrolGains.P_VZ  I=VTOLcontrolGains.I_VZ  UseKiTs=off  D=VTOLcontrolGains.D_VZ  UseExternalDerivativeSource=off  N=VTOLcontrolGains.N_VZ  UseFilter=on  TunerSelectOption=Transfer Function Based (PID Tuner App)  InitialConditionSource=internal  InitialConditionForIntegrator=0  InitialConditionForFilter=0  DifferentiatorICPrevScaledInput=0  ExternalReset=level  TrackingMode=off  Kt=1  LimitOutput=off  SatLimitsSource=internal  UpperSaturationLimit=inf  LowerSaturationLimit=-inf  LinearizeAsGain=on  AntiWindupMode=none  Kb=1  LimitIntegrator=off  UpperIntegratorSaturationLimit=inf  LowerIntegratorSaturationLimit=-inf  POutMin=[]  POutMax=[]  IOutMin=[]  IOutMax=[]  DOutMin=[]  DOutMax=[]  NOutMin=[]  NOutMax=[]  SumOutMin=[]  SumOutMax=[]  SaturationOutMin=[]  SaturationOutMax=[]  PParamMin=[]  PParamMax=[]  IParamMin=[]  IParamMax=[]  DParamMin=[]  DParamMax=[]  NParamMin=[]  NParamMax=[]  KbParamMin=[]  KbParamMax=[]  KtParamMin=[]  KtParamMax=[]  KbOutMin=[]  KbOutMax=[]  KtOutMin=[]  KtOutMax=[]  IntegratorOutMin=[]  IntegratorOutMax=[]  FilterOutMin=[]  FilterOutMax=[]  SumI1OutMin=[]  SumI1OutMax=[]  SumI2OutMin=[]  SumI2OutMax=[]  SumI3OutMin=[]  SumI3OutMax=[]  SumI4OutMin=[]  SumI4OutMax=[]  SumDOutMin=[]  SumDOutMax=[]  DifferentiatorOutMin=[]  DifferentiatorOutMax=[]  FilterDiffOutCoefMin=[]  FilterDiffOutCoefMax=[]  ReciprocalOutMin=[]  ReciprocalOutMax=[]  SumDenOutMin=[]  SumDenOutMax=[]  SumNumOutMin=[]  SumNumOutMax=[]  DivideOutMin=[]  DivideOutMax=[]  UdiffTsProdOutMin=[]  UdiffTsProdOutMax=[]  NTsProdOutMin=[]  NTsProdOutMax=[]  UintegralTsProdOutMin=[]  UintegralTsProdOutMax=[]  UngainTsProdOutMin=[]  UngainTsProdOutMax=[]  ClampingZeroOutDataTypeStr=Inherit: Inherit via back propagation  ClampingZeroOutMin=[]  ClampingZeroOutMax=[]  FilterDenConstantOutDataTypeStr=Inherit: Inherit via back propagation  FilterDenConstantOutMin=[]  FilterDenConstantOutMax=[]  PCopyOutDataTypeStr=Inherit: Inherit via back propagation  PCopyOutMin=[]  PCopyOutMax=[]  NCopyOutDataTypeStr=Inherit: Inherit via back propagation  NCopyOutMin=[]  NCopyOutMax=[]  IntegratorContinuousStateAttributes=''  IntegratorStateMustResolveToSignalObject=off  IntegratorRTWStateStorageClass=Auto  FilterContinuousStateAttributes=''  FilterStateMustResolveToSignalObject=off  FilterRTWStateStorageClass=Auto  ParallelPVariant=InternalParameters  IdealPVariant=Disabled  IVariant=InternalParameters  DVariant=InternalParameters  IntegratorVariant=Discrete  SatVariant=Disabled  AWVariant=Passthrough  PCopyVariant=Disabled  TRVariant=Disabled  FdbkBlocksVariant=Forward  IdealPFdbkVariant=Disabled  SatFdbkVariant=Disabled  DerivativeFilterVariant=ForwardEulerFilter  NVariant=InternalParameters  NCopyVariant=Disabled  FilterICVariant=InternalICsFilter  IntegratorICVariant=InternalICs  ExternalResetVariant=ExternalReset  TRSumVariant=Passthrough  SumFdbkVariant=Disabled  SumVariant=Sum_PID  TsampFilterVariant=InternalTs  TsampNgainVariant=Passthrough  TsampIntegralVariant=Disabled_SignalSpec  ExternalSaturationOutDataTypeStr=Inherit: Same as second input  DerivativeSourceVariant=ErrorSignal  PreIntVariant=InternalPreInt
  Bus Selector : BusSelector  OutputSignals=Xe,Ve
  Constant1 : Constant  Value=flightState.Transition
  Constant2 : Constant  Value=flightState.BackTransition
  Constant3 : Constant  Value=flightState.Hover
  Constant4 : Constant  Value=flightState.FixedWing
  Equal{,1..3} (4 alike) : RelationalOperator  Operator===  OutDataTypeStr=boolean  RndMeth=Simplest  InputSameDT=off
  Gain : Gain  Gain=-1
  Logical Operator : Logic  Operator=OR  AllPortsSameDT=off  OutDataTypeStr=boolean
  Logical Operator1 : Logic  Operator=OR  AllPortsSameDT=off  OutDataTypeStr=boolean
  Logical Operator2 : Logic  Operator=NOT  AllPortsSameDT=off  OutDataTypeStr=boolean
  NOT : Logic  Operator=NOT  IconShape=distinctive  AllPortsSameDT=off  OutDataTypeStr=boolean
  Rate Limiter : RateLimiter  RisingSlewLimit=controlParams.VTOLmaxAltErrratelimit  FallingSlewLimit=controlParams.VTOLminAltErrratelimit  SampleTimeMode=inherited
  Saturation : Saturate  UpperLimit=controlParams.VTOLmaxVerticalSPD  LowerLimit=controlParams.VTOLminVerticalSPD
  Selector : Selector  InputPortWidth=3  IndexOptions=Index vector (dialog)  Indices=[3]  OutputSizes=1
  Selector1 : Selector  InputPortWidth=3  IndexOptions=Index vector (dialog)  Indices=[3]  OutputSizes=1
  Sum : Sum  Inputs=|+-
  Sum1 : Sum  Inputs=|+-
  Switch : Switch  Criteria=u2 > Threshold  SaturateOnIntegerOverflow=off  InputSameDT=off
  Switch1 : Switch  Criteria=u2 > Threshold  SaturateOnIntegerOverflow=off  InputSameDT=off
  Triggered Subsystem : Subsystem  TreatAsAtomicUnit=on
  commanded thrust : Outport
  wires:
  States/1 -> Bus Selector/1
  InTransition/1 -> NOT/1, Triggered Subsystem/Trigger
  Switch/1 -> Sum/1  "Output"
  NOT/1 -> Switch/2
  Triggered Subsystem/1(Reference) -> [AltHoldCmd]  "Stable"
  Selector/1 -> Alt signal condition/1(Z_in), Triggered Subsystem/1(AltHold)
  Bus Selector/1 -> Selector/1  "<Xe>"
  Bus Selector/2 -> Selector1/1  "<Ve>"
  Sum1/1 -> Altitude rate controller/1
  Alt signal condition/1(Z_out) -> Sum/2
  Constant4/1 -> Equal/1
  Equal/1 -> Switch1/2
  Z ref/1 -> Switch1/3  "Manual"
  Switch1/1 -> Switch/1  "Output"
  Sum/1 -> Rate Limiter/1
  Selector1/1 -> Sum1/2
  Altitude rate controller/1 -> Gain/1  "Output"
  Gain/1 -> commanded thrust/1
  [AltHoldCmd] -> Switch1/1
  [AltHoldCmd] -> Switch/3
  Saturation/1 -> Sum1/1
  Altitude controller/1 -> Saturation/1
  Rate Limiter/1 -> Altitude controller/1
  Equal1/1 -> Logical Operator/1
  Equal2/1 -> Logical Operator/2
  Logical Operator2/1 -> [int_reset]
  Constant2/1 -> Equal3/1
  Constant3/1 -> Equal1/1
  FlightMode/1 -> Equal1/2, Equal2/2, Equal3/2, Equal/2
  Equal3/1 -> Logical Operator1/2
  Logical Operator/1 -> Logical Operator1/1
  Logical Operator1/1 -> Logical Operator2/1
  Constant1/1 -> Equal2/1
  [int_reset] -> Altitude rate controller/2
